simulink model "sampleModel2438_pp"  (R2018a)
settings: Solver=VariableStepAuto  StartTime=0.0  StopTime=10.0  RelTol=1e-3
undefined symbols (not defined in the file or in its folder): DiscIntNeverNeededParam, sigbuilder_block
libraries: simulink x299
(part 1 of 6)
settings Model: Creator=cyfuzz  LastModifiedBy=shafiul
settings CodeAppCC: StateflowObjectComments=on

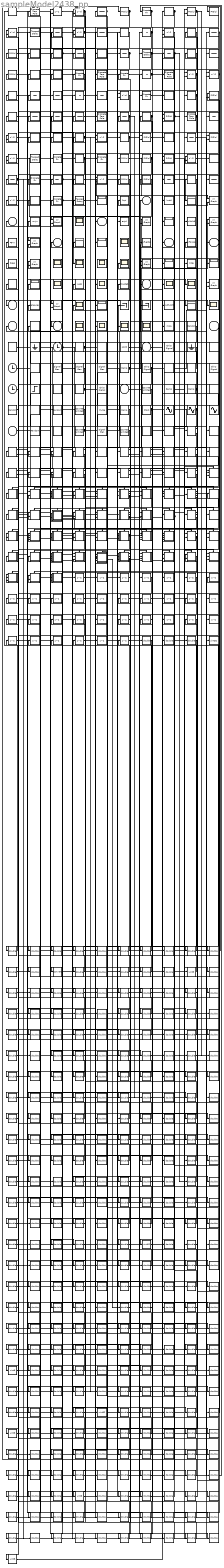
== system sampleModel2438_pp ==
  cfblk160 : Inport
  cfblk167 : Inport  Port=2
  cfblk186 : Inport  Port=3
  cfblk201 : Inport  Port=4
  cfblk{1,32,64,66,74,80,92} (7 alike) : simulink/Discrete/Transfer Fcn Real Zero  ZeroZ=0.75  ICPrevInput=0.0  DoSatur=off
      settings: SourceProductName=Simulink  SourceProductBaseCode=SL
  cfblk{6,10,21,31,76..77,86..87} (8 alike) : simulink/Continuous/PID Controller  Controller=PID  TimeDomain=Discrete-time  SampleTime=1  IntegratorMethod=Forward Euler  FilterMethod=Forward Euler  Form=Parallel  UseFilter=on  ControllerParametersSource=internal  P=1  I=1  D=0  N=100  InitialConditionSource=internal  InitialConditionForIntegrator=0  InitialConditionForFilter=0  ExternalReset=none  LimitOutput=off  UpperSaturationLimit=inf  LowerSaturationLimit=-inf  LinearizeAsGain=off  AntiWindupMode=none  Kb=1  TrackingMode=off  Kt=1  PParamMin=[]  PParamMax=[]  IParamMin=[]  IParamMax=[]  DParamMin=[]  DParamMax=[]  NParamMin=[]  NParamMax=[]  KbParamMin=[]  KbParamMax=[]  KtParamMin=[]  KtParamMax=[]  POutMin=[]  POutMax=[]  IOutMin=[]  IOutMax=[]  DOutMin=[]  DOutMax=[]  NOutMin=[]  NOutMax=[]  KbOutMin=[]  KbOutMax=[]  KtOutMin=[]  KtOutMax=[]  IntegratorOutMin=[]  IntegratorOutMax=[]  FilterOutMin=[]  FilterOutMax=[]  SumOutMin=[]  SumOutMax=[]  SumI1OutMin=[]  SumI1OutMax=[]  SumI2OutMin=[]  SumI2OutMax=[]  SumI3OutMin=[]  SumI3OutMax=[]  SumDOutMin=[]  SumDOutMax=[]  SaturationOutMin=[]  SaturationOutMax=[]  IntegratorContinuousStateAttributes=''  IntegratorStateMustResolveToSignalObject=off  IntegratorRTWStateStorageClass=Auto  FilterContinuousStateAttributes=''  FilterStateMustResolveToSignalObject=off  FilterRTWStateStorageClass=Auto  DifferentiatorICPrevScaledInput=0  DifferentiatorOutMin=[]  DifferentiatorOutMax=[]  FilterDiffOutCoefMin=[]  FilterDiffOutCoefMax=[]  SumDenOutMin=[]  SumDenOutMax=[]  SumNumOutMin=[]  SumNumOutMax=[]  ReciprocalOutMin=[]  ReciprocalOutMax=[]  DivideOutMin=[]  DivideOutMax=[]  TunerSelectOption=Transfer Function Based (PID Tuner App)
  cfblk{100,103,107,110,112,122,127,140,143} (9 alike) : simulink/Sinks/XY Graph  xmin=-1  xmax=1  ymin=-1  ymax=1  st=-1
  cfblk102 : ToFile  Filename=mvju  SaveFormat=Timeseries
  cfblk{104,116,123..126,133,135,138..139,144,150,154..157} (16 alike) : Scope
      cfblk104 settings: Floating=on
      cfblk116 settings: Floating=on
      cfblk123 settings: Floating=on
      cfblk125 settings: Floating=on
      cfblk133 settings: Floating=on
      cfblk154 settings: Floating=on
      cfblk157 settings: Floating=on
  cfblk106 : ToFile  Filename=eujd  SaveFormat=Timeseries
  cfblk{95,99,108,114..115,128,130,132,145,149} (10 alike) : Display
  cfblk109 : ToWorkspace  VariableName=xkbihtf  SaveFormat=Timeseries  SampleTime=-1
  cfblk11 : Delay  DelayLengthSource=Input port  SampleTime=1
      settings: InputPortMap=u0,p1
  cfblk111 : ToFile  Filename=cgvy  SaveFormat=Timeseries
  cfblk117 : ToWorkspace  VariableName=xfyezbp  SaveFormat=Timeseries  SampleTime=-1
  cfblk119 : ToWorkspace  VariableName=yrfonpq  SaveFormat=Timeseries  SampleTime=-1
  cfblk{12,27,72,94} (4 alike) : simulink/Discrete/Tapped Delay  vinit=0.0  samptime=-1  NumDelays=1  DelayOrder=Oldest  includeCurrent=off
  cfblk121 : ToFile  Filename=bcgq  SaveFormat=Timeseries
  cfblk129 : ToFile  Filename=mjtg  SaveFormat=Timeseries
  cfblk{13,15,20,43,52..53,56,81,90} (9 alike) : DiscreteTransferFcn  SampleTime=1
  cfblk131 : ToWorkspace  VariableName=whweswj  SaveFormat=Timeseries  SampleTime=-1
  cfblk134 : ToFile  Filename=jueb  SaveFormat=Timeseries
  cfblk136 : ToWorkspace  VariableName=tkwpteb  SaveFormat=Timeseries  SampleTime=-1
  cfblk{3,14,18,39..40,61,65,71,79,85} (10 alike) : Delay  ShowEnablePort=on  SampleTime=1
      settings: InputPortMap=u0,e6
  cfblk142 : ToWorkspace  VariableName=enguigy  SaveFormat=Timeseries  SampleTime=-1
  cfblk146 : Terminator
  cfblk147 : Terminator
  cfblk148 : ToWorkspace  VariableName=wdhubit  SaveFormat=Timeseries  SampleTime=-1
  cfblk152 : ToWorkspace  VariableName=eyoxfmy  SaveFormat=Timeseries  SampleTime=-1
  cfblk158 : ToFile  Filename=mojy  SaveFormat=Timeseries
  cfblk{159,191,193,202} (4 alike) : UniformRandomNumber  SampleTime=0.1
  cfblk16 : simulink/Discrete/Transfer Fcn Lead or Lag  PoleZ=0.95  ZeroZ=0.75  ICPrevOutput=0.0  ICPrevInput=0.0  DoSatur=off
      settings: SourceProductName=Simulink  SourceProductBaseCode=SL
  cfblk161 : simulink/Sources/Band-Limited White Noise  Cov=[0.1]  Ts=0.1  seed=[23341]
  cfblk162 : Ground
  cfblk163 : Clock
  cfblk164 : simulink/Sources/Band-Limited White Noise  Cov=[0.1]  Ts=0.1  seed=[23341]
  cfblk165 : Subsystem  Tag=STV Subsys  LoadFcn=sigbuilder_block('load');  StartFcn=sigbuilder_block('start');  StopFcn=sigbuilder_block('stop');  ClipboardFcn=sigbuilder_block('clipboard');  mask(Sigbuilder block){tuvar=[0:10]}
      mask help: Simulink:masks:SigbuilderBlock_MD
      mask init:
      | if ~strcmp(get_param(bdroot(gcbh),'SimulationStatus'),'stopped') tuvar = sigbuilder_block('maskInit'); end
      settings: CopyFcn=sigbuilder_block('copy');  DeleteFcn=sigbuilder_block('delete');  ModelCloseFcn=sigbuilder_block('modelClose');  PreSaveFcn=sigbuilder_block('preSave');  PauseFcn=sigbuilder_block('pause');  ContinueFcn=sigbuilder_block('continue');  NameChangeFcn=sigbuilder_block('namechange');  OpenFcn=sigbuilder_block('open',[437.6 199.2 550.4 400 ]);  CloseFcn=sigbuilder_block('close');
      mask Display: plot(0, 0, 100, 100,[2, 2, 32, 32, 2], [68, 8, 8, 68, 68],[32, 2], [38, 38], [32, 19, 2],[53, 60, 44], [32, 17, 17, 2],[16, 16, 31, 31]);txt = getActiveGroup(gcbh);text(2, 100, txt,'verticalAlignment', 'top');
  cfblk166 : Constant  Value=4120
  cfblk{168,177,180,185} (4 alike) : simulink/Sources/Chirp Signal  f1=0.1  T=100  f2=1
  cfblk169 : Ground
  cfblk17 : UnitDelay
  cfblk170 : Subsystem  Tag=STV Subsys  LoadFcn=sigbuilder_block('load');  StartFcn=sigbuilder_block('start');  StopFcn=sigbuilder_block('stop');  ClipboardFcn=sigbuilder_block('clipboard');  mask(Sigbuilder block){tuvar=[0:10]}
      mask help: Simulink:masks:SigbuilderBlock_MD
      mask init:
      | if ~strcmp(get_param(bdroot(gcbh),'SimulationStatus'),'stopped') tuvar = sigbuilder_block('maskInit'); end
      settings: CopyFcn=sigbuilder_block('copy');  DeleteFcn=sigbuilder_block('delete');  ModelCloseFcn=sigbuilder_block('modelClose');  PreSaveFcn=sigbuilder_block('preSave');  PauseFcn=sigbuilder_block('pause');  ContinueFcn=sigbuilder_block('continue');  NameChangeFcn=sigbuilder_block('namechange');  OpenFcn=sigbuilder_block('open',[437.6 199.2 550.4 400 ]);  CloseFcn=sigbuilder_block('close');
      mask Display: plot(0, 0, 100, 100,[2, 2, 32, 32, 2], [68, 8, 8, 68, 68],[32, 2], [38, 38], [32, 19, 2],[53, 60, 44], [32, 17, 17, 2],[16, 16, 31, 31]);txt = getActiveGroup(gcbh);text(2, 100, txt,'verticalAlignment', 'top');
  cfblk171 : Clock
  cfblk{172,178,190,192} (4 alike) : simulink/Sources/Repeating Sequence  rep_seq_t=[0 2]  rep_seq_y=[0 2]
  cfblk{173..175,205} (4 alike) : SignalGenerator  Units=rad/sec
  cfblk{176,188..189,196} (4 alike) : simulink/Sources/Ramp  slope=1  start=0  InitialOutput=0
  cfblk179 : Subsystem  Tag=STV Subsys  LoadFcn=sigbuilder_block('load');  StartFcn=sigbuilder_block('start');  StopFcn=sigbuilder_block('stop');  ClipboardFcn=sigbuilder_block('clipboard');  mask(Sigbuilder block){tuvar=[0:10]}
      mask help: Simulink:masks:SigbuilderBlock_MD
      mask init:
      | if ~strcmp(get_param(bdroot(gcbh),'SimulationStatus'),'stopped') tuvar = sigbuilder_block('maskInit'); end
      settings: CopyFcn=sigbuilder_block('copy');  DeleteFcn=sigbuilder_block('delete');  ModelCloseFcn=sigbuilder_block('modelClose');  PreSaveFcn=sigbuilder_block('preSave');  PauseFcn=sigbuilder_block('pause');  ContinueFcn=sigbuilder_block('continue');  NameChangeFcn=sigbuilder_block('namechange');  OpenFcn=sigbuilder_block('open',[437.6 199.2 550.4 400 ]);  CloseFcn=sigbuilder_block('close');
      mask Display: plot(0, 0, 100, 100,[2, 2, 32, 32, 2], [68, 8, 8, 68, 68],[32, 2], [38, 38], [32, 19, 2],[53, 60, 44], [32, 17, 17, 2],[16, 16, 31, 31]);txt = getActiveGroup(gcbh);text(2, 100, txt,'verticalAlignment', 'top');
  cfblk181 : Clock
  cfblk182 : Step  After=81  SampleTime=0
  cfblk183 : simulink/Sources/Repeating Sequence Stair  OutValues=[3 1 4 2 1].'  tsamp=-1  OutMin=[]  OutMax=[]  OutDataTypeStr=double  OutputDataTypeScalingMode=double  OutDataType=fixdt(0,8)  ConRadixGroup=Best Precision: Vector-wise  OutScaling=2^-12
  cfblk184 : simulink/Sources/Repeating Sequence Interpolated  OutValues=[3 1 4 2 1].'  TimeValues=[0 0.1 0.5 0.6 1].'  LookUpMeth=Interpolation-Use End Values  tsamp=0.01  OutMin=[]  OutMax=[]  OutDataTypeStr=double  OutputDataTypeScalingMode=double  OutDataType=fixdt(0,8)  OutScaling=2^-10
  cfblk{187,194,204,206} (4 alike) : simulink/Sources/Counter Limited  uplimit=7  tsamp=-1
  cfblk{8,19,23,48} (4 alike) : DiscreteStateSpace
  cfblk195 : DiscretePulseGenerator  PulseType=Time based  Period=10  PulseWidth=5
  cfblk197 : DigitalClock
  cfblk198 : Sin  SampleTime=0
  cfblk199 : Sin  SampleTime=0
  cfblk{2,35,38,55,59} (5 alike) : DiscreteZeroPole  Poles=[0 0.5]  Gain=1
  cfblk200 : Sin  SampleTime=0
  cfblk203 : simulink/Sources/Band-Limited White Noise  Cov=[0.1]  Ts=0.1  seed=[23341]
  cfblk207 : Subsystem  Tag=STV Subsys  LoadFcn=sigbuilder_block('load');  StartFcn=sigbuilder_block('start');  StopFcn=sigbuilder_block('stop');  ClipboardFcn=sigbuilder_block('clipboard');  mask(Sigbuilder block){tuvar=[0:10]}
      mask help: Simulink:masks:SigbuilderBlock_MD
      mask init:
      | if ~strcmp(get_param(bdroot(gcbh),'SimulationStatus'),'stopped') tuvar = sigbuilder_block('maskInit'); end
      settings: CopyFcn=sigbuilder_block('copy');  DeleteFcn=sigbuilder_block('delete');  ModelCloseFcn=sigbuilder_block('modelClose');  PreSaveFcn=sigbuilder_block('preSave');  PauseFcn=sigbuilder_block('pause');  ContinueFcn=sigbuilder_block('continue');  NameChangeFcn=sigbuilder_block('namechange');  OpenFcn=sigbuilder_block('open',[437.6 199.2 550.4 400 ]);  CloseFcn=sigbuilder_block('close');
      mask Display: plot(0, 0, 100, 100,[2, 2, 32, 32, 2], [68, 8, 8, 68, 68],[32, 2], [38, 38], [32, 19, 2],[53, 60, 44], [32, 17, 17, 2],[16, 16, 31, 31]);txt = getActiveGroup(gcbh);text(2, 100, txt,'verticalAlignment', 'top');
  cfblk{208..229} (22 alike) : If  SampleTime=1
  cfblk{22,33,63,89} (4 alike) : simulink/Discrete/Transfer Fcn First Order  PoleZ=0.95  ICPrevOutput=0.0  DoSatur=off
      settings: SourceProductName=Simulink
  cfblk230 : Subsystem  TreatAsAtomicUnit=on
  cfblk231 : Subsystem  TreatAsAtomicUnit=on
  cfblk232 : Subsystem  TreatAsAtomicUnit=on
  cfblk233 : Subsystem  TreatAsAtomicUnit=on
  cfblk234 : Subsystem  TreatAsAtomicUnit=on
  cfblk235 : Subsystem  TreatAsAtomicUnit=on
  cfblk236 : Subsystem  TreatAsAtomicUnit=on
  cfblk237 : Subsystem  TreatAsAtomicUnit=on
  cfblk238 : Subsystem  TreatAsAtomicUnit=on
  cfblk239 : Subsystem  TreatAsAtomicUnit=on
  cfblk{5,24,30,54} (4 alike) : DiscreteFilter  SampleTime=1
  cfblk240 : Subsystem  TreatAsAtomicUnit=on
  cfblk241 : Subsystem  TreatAsAtomicUnit=on
  cfblk242 : Subsystem  TreatAsAtomicUnit=on
  cfblk243 : Subsystem  TreatAsAtomicUnit=on
  cfblk244 : Subsystem  TreatAsAtomicUnit=on
  cfblk245 : Subsystem  TreatAsAtomicUnit=on
  cfblk246 : Subsystem  TreatAsAtomicUnit=on
  cfblk247 : Subsystem  TreatAsAtomicUnit=on
  cfblk248 : Subsystem  TreatAsAtomicUnit=on
  cfblk249 : Subsystem  TreatAsAtomicUnit=on
  cfblk{25,29,41,57,62,68,84} (7 alike) : simulink/Discrete/Difference  ICPrevInput=0.0  OutMin=[]  OutMax=[]  OutDataTypeStr=Inherit: Inherit via back propagation  OutDataType=fixdt(1, 16)  OutScaling=2^-10  DoSatur=off
  cfblk250 : Subsystem  TreatAsAtomicUnit=on
  cfblk251 : Subsystem  TreatAsAtomicUnit=on
  cfblk252 : Subsystem  TreatAsAtomicUnit=on
  cfblk253 : Subsystem  TreatAsAtomicUnit=on
  cfblk254 : Subsystem  TreatAsAtomicUnit=on
  cfblk255 : Subsystem  TreatAsAtomicUnit=on
  cfblk256 : Subsystem  TreatAsAtomicUnit=on
  cfblk257 : Subsystem  TreatAsAtomicUnit=on
  cfblk258 : Subsystem  TreatAsAtomicUnit=on
  cfblk259 : Subsystem  TreatAsAtomicUnit=on
  cfblk{26,28,42,45,60,69,83,88} (8 alike) : DiscreteIntegrator  ICPrevOutput=DiscIntNeverNeededParam  ICPrevScaledInput=DiscIntNeverNeededParam
  cfblk260 : Subsystem  TreatAsAtomicUnit=on
  cfblk261 : Subsystem  TreatAsAtomicUnit=on
  cfblk262 : Subsystem  TreatAsAtomicUnit=on
  cfblk263 : Subsystem  TreatAsAtomicUnit=on
  cfblk264 : Subsystem  TreatAsAtomicUnit=on
  cfblk265 : Subsystem  TreatAsAtomicUnit=on
  cfblk266 : Subsystem  TreatAsAtomicUnit=on
  cfblk267 : Subsystem  TreatAsAtomicUnit=on
  cfblk268 : Subsystem  TreatAsAtomicUnit=on
  cfblk269 : Subsystem  TreatAsAtomicUnit=on
  cfblk270 : Subsystem  TreatAsAtomicUnit=on
  cfblk271 : Subsystem  TreatAsAtomicUnit=on
  cfblk272 : Subsystem  TreatAsAtomicUnit=on
  cfblk273 : Subsystem  TreatAsAtomicUnit=on
  cfblk{91,274..306} (34 alike) : Delay  SampleTime=1
  cfblk307 : DataTypeConversion  OutDataTypeStr=double
  cfblk308 : DataTypeConversion  OutDataTypeStr=double
  cfblk309 : DataTypeConversion  OutDataTypeStr=double
  cfblk310 : DataTypeConversion  OutDataTypeStr=uint32
  cfblk{7,34,36,47,73,75,82,93} (8 alike) : DiscreteFir  SampleTime=1
  cfblk37 : UnitDelay
  cfblk4 : Delay  DelayLengthSource=Input port  SampleTime=1
      settings: InputPortMap=u0,p1
  cfblk44 : UnitDelay
  cfblk46 : Delay  DelayLengthSource=Input port  SampleTime=1
      settings: InputPortMap=u0,p1
  cfblk49 : simulink/Discrete/Transfer Fcn Lead or Lag  PoleZ=0.95  ZeroZ=0.75  ICPrevOutput=0.0  ICPrevInput=0.0  DoSatur=off
      settings: SourceProductName=Simulink  SourceProductBaseCode=SL
  cfblk{9,50,58,67,70,78} (6 alike) : simulink/Continuous/PID Controller (2DOF)  Controller=PID  TimeDomain=Discrete-time  SampleTime=1  IntegratorMethod=Forward Euler  FilterMethod=Forward Euler  Form=Parallel  UseFilter=on  ControllerParametersSource=internal  P=1  I=1  D=0  N=100  b=1  c=1  InitialConditionSource=internal  InitialConditionForIntegrator=0  InitialConditionForFilter=0  ExternalReset=none  LimitOutput=off  UpperSaturationLimit=inf  LowerSaturationLimit=-inf  LinearizeAsGain=off  AntiWindupMode=none  Kb=1  TrackingMode=off  Kt=1  PParamMin=[]  PParamMax=[]  IParamMin=[]  IParamMax=[]  DParamMin=[]  DParamMax=[]  NParamMin=[]  NParamMax=[]  bParamMin=[]  bParamMax=[]  cParamMin=[]  cParamMax=[]  KbParamMin=[]  KbParamMax=[]  KtParamMin=[]  KtParamMax=[]  POutMin=[]  POutMax=[]  IOutMin=[]  IOutMax=[]  DOutMin=[]  DOutMax=[]  NOutMin=[]  NOutMax=[]  bOutMin=[]  bOutMax=[]  cOutMin=[]  cOutMax=[]  KbOutMin=[]  KbOutMax=[]  KtOutMin=[]  KtOutMax=[]  IntegratorOutMin=[]  IntegratorOutMax=[]  FilterOutMin=[]  FilterOutMax=[]  SumOutMin=[]  SumOutMax=[]  Sum1OutMin=[]  Sum1OutMax=[]  Sum2OutMin=[]  Sum2OutMax=[]  Sum3OutMin=[]  Sum3OutMax=[]  SumI1OutMin=[]  SumI1OutMax=[]  SumI2OutMin=[]  SumI2OutMax=[]  SumI3OutMin=[]  SumI3OutMax=[]  SumDOutMin=[]  SumDOutMax=[]  SaturationOutMin=[]  SaturationOutMax=[]  IntegratorContinuousStateAttributes=''  IntegratorStateMustResolveToSignalObject=off  IntegratorRTWStateStorageClass=Auto  FilterContinuousStateAttributes=''  FilterStateMustResolveToSignalObject=off  FilterRTWStateStorageClass=Auto  DifferentiatorICPrevScaledInput=0  DifferentiatorOutMin=[]  DifferentiatorOutMax=[]  FilterDiffOutCoefMin=[]  FilterDiffOutCoefMax=[]  SumDenOutMin=[]  SumDenOutMax=[]  SumNumOutMin=[]  SumNumOutMax=[]  ReciprocalOutMin=[]  ReciprocalOutMax=[]  DivideOutMin=[]  DivideOutMax=[]  TunerSelectOption=Transfer Function Based (PID Tuner App)
  cfblk51 : simulink/Discrete/Transfer Fcn Lead or Lag  PoleZ=0.95  ZeroZ=0.75  ICPrevOutput=0.0  ICPrevInput=0.0  DoSatur=off
      settings: SourceProductName=Simulink  SourceProductBaseCode=SL
  cfblk96 : ToFile  Filename=fnpi  SaveFormat=Timeseries
  cfblk98 : ToFile  Filename=kudd  SaveFormat=Timeseries
  cyemi_{0..11,13..17,19..58,72,83..84,111..113,128..129,175..177,213..214,223..224,233..235,251,309..310,318,347..348,360..361,375..376,383..385,414,450..451,472,508,513..514,524..525,534..537,550..551,569..570,598..599,608..610,651..654,700..703,775..776,783..785,796,807,851..854,859..861,865..869,873..875,924..927,938,946..947,956..959,1005..1007,1014..1015,1026..1028,1037..1074,1076..1098,1100..1104,1106..1137,1139..1164} (283 alike) : DataTypeConversion  OutDataTypeStr=double
  cyemi_{18,1075,1105,1138,1165} (5 alike) : DataTypeConversion  OutDataTypeStr=uint8
  cyemi_1099 : DataTypeConversion  OutDataTypeStr=uint32
  cyemi_12 : DataTypeConversion  OutDataTypeStr=fixdt('ufix32_En8')
  cyemi_937 : DataTypeConversion  OutDataTypeStr=uint32
  cfblk97 : Outport
  cfblk101 : Outport  Port=2
  cfblk105 : Outport  Port=3
  cfblk113 : Outport  Port=4
  cfblk118 : Outport  Port=5
  cfblk120 : Outport  Port=6
  cfblk137 : Outport  Port=7
  cfblk141 : Outport  Port=8
  cfblk151 : Outport  Port=9
  cfblk153 : Outport  Port=10
  wires:
  cfblk10/1 -> cfblk135/1
  cfblk200/1 -> cfblk108/1
  cfblk83/1 -> cyemi_703/1, cyemi_1121/1
  cfblk58/1 -> cyemi_58/1, cyemi_1055/1, cyemi_1157/1
  cfblk45/1 -> cfblk145/1
  cfblk16/1 -> cfblk155/1
  cfblk4/1 -> cyemi_1058/1, cyemi_1155/1
  cfblk52/1 -> cfblk124/1
  cfblk23/1 -> cyemi_700/1, cyemi_1129/1
  cfblk189/1 -> cfblk118/1, cyemi_654/1, cyemi_1005/1
  cfblk195/1 -> cfblk97/1
  cfblk230/1(cfblk2) -> cfblk126/1, cyemi_1056/1
  cfblk176/1 -> cfblk107/1, cyemi_57/1
  cfblk15/1 -> cfblk147/1, cyemi_1113/1
  cfblk14/1 -> cyemi_29/1, cyemi_861/1
  cfblk77/1 -> cyemi_550/1, cyemi_1006/1
  cfblk199/1 -> cyemi_14/1, cyemi_234/1
  cfblk87/1 -> cfblk103/1
  cfblk62/1 -> cfblk149/1
  cfblk57/1 -> cfblk143/1, cyemi_3/1, cyemi_1057/1, cyemi_1125/1
  cfblk6/1 -> cfblk143/2, cfblk105/1
  cfblk244/1(cfblk2) -> cyemi_52/1, cyemi_1092/1
  cfblk55/1 -> cyemi_4/1, cyemi_1109/1
  cfblk84/1 -> cfblk100/1
  cfblk91/1 -> cfblk103/2
  cfblk24/1 -> cfblk112/1
  cfblk90/1 -> cfblk127/1
  cfblk8/1 -> cyemi_860/1, cyemi_1051/1
  cfblk197/1 -> cyemi_30/1, cyemi_1084/1
  cfblk59/1 -> cyemi_1079/1, cyemi_1096/1
  cfblk163/1 -> cyemi_41/1, cyemi_514/1
  cfblk20/1 -> cyemi_177/1, cyemi_785/1
  cfblk205/1 -> cfblk140/2, cyemi_1102/1
  cfblk204/1 -> cfblk146/1, cyemi_18/1, cyemi_1138/1
  cfblk86/1 -> cfblk141/1
  cfblk240/2(cfblk8) -> cyemi_869/1, cyemi_1073/1
  cfblk74/1 -> cyemi_55/1, cyemi_854/1
  cfblk28/1 -> cyemi_702/1, cyemi_1146/1
  cfblk66/1 -> cyemi_24/1, cyemi_1163/1
  cfblk177/1 -> cyemi_1/1, cyemi_1043/1
  cfblk40/1 -> cyemi_49/1, cyemi_1074/1
  cfblk250/1(cfblk2) -> cfblk128/1
  cfblk246/3(cfblk10) -> cfblk138/1, cyemi_1070/1
  cfblk255/1(cfblk2) -> cfblk101/1
  cfblk11/1 -> cfblk139/1
  cfblk261/2(cfblk11) -> cyemi_957/1, cyemi_1156/1
  cfblk256/1(cfblk2) -> cfblk110/1, cyemi_1135/1
  cfblk182/1 -> cfblk112/2
  cfblk264/1(cfblk2) -> cfblk114/1
  cfblk257/1(cfblk2) -> cfblk151/1, cyemi_36/1
  cfblk81/1 -> cyemi_21/1, cyemi_25/1
  cfblk27/1 -> cyemi_385/1, cyemi_958/1
  cfblk85/1 -> cfblk156/1
  cfblk37/1 -> cfblk150/1, cyemi_1015/1
  cfblk248/2(cfblk11) -> cyemi_1067/1, cyemi_1077/1
  cfblk12/1 -> cfblk95/1
  cfblk93/1 -> cfblk107/2, cyemi_701/1
  cfblk201/1 -> cfblk120/1
  cfblk71/1 -> cfblk115/1
  cfblk64/1 -> cyemi_5/1, cyemi_1089/1
  cfblk259/2(cfblk8) -> cyemi_213/1, cyemi_938/1
  cfblk5/1 -> cyemi_536/1, cyemi_1068/1
  cfblk245/1(cfblk2) -> cfblk122/1, cyemi_853/1
  cfblk184/1 -> cfblk130/1, cyemi_27/1, cyemi_43/1
  cfblk232/1(cfblk2) -> cyemi_1090/1, cyemi_1143/1
  cfblk179/1(Signal 1) -> cfblk132/1
  cfblk48/1 -> cfblk122/2
  cfblk160/1 -> cyemi_214/1, cyemi_867/1
  cfblk76/1 -> cfblk99/1
  cfblk26/1 -> cyemi_472/1, cyemi_959/1
  cfblk7/1 -> cyemi_44/1, cyemi_610/1
  cfblk39/1 -> cfblk127/2, cyemi_1119/1
  cfblk49/1 -> cyemi_53/1, cyemi_537/1
  cfblk88/1 -> cfblk110/2
  cfblk9/1 -> cyemi_72/1, cyemi_1053/1
  cfblk265/2(cfblk10) -> cyemi_1049/1, cyemi_1050/1
  cfblk162/1 -> cyemi_54/1, cyemi_383/1
  cfblk272/1(cfblk2) -> cyemi_513/1, cyemi_868/1
  cfblk203/1 -> cfblk113/1
  cfblk17/1 -> cyemi_551/1, cyemi_926/1
  cfblk238/2(cfblk17) -> cfblk100/2
  cfblk164/1 -> cyemi_1080/1, cyemi_1152/1
  cfblk235/2(cfblk12) -> cfblk144/1
  cfblk44/1 -> cfblk137/1
  cfblk56/1 -> cfblk153/1, cyemi_235/1
  cfblk266/3(cfblk16) -> cyemi_1054/1, cyemi_1118/1
  cfblk260/3(cfblk15) -> cyemi_26/1, cyemi_1145/1
  cfblk178/1 -> cfblk140/1
  cfblk170/1(Signal 1) -> cyemi_6/1, cyemi_23/1, cyemi_28/1
  cfblk234/3(cfblk15) -> cyemi_1039/1, cyemi_1101/1
  cfblk236/3(cfblk12) -> cyemi_1088/1, cyemi_1103/1
  cfblk208/1 -> cfblk230/Action
  cfblk208/2 -> cfblk231/Action
  cfblk209/1 -> cfblk232/Action
  cfblk209/2 -> cfblk233/Action
  cfblk210/1 -> cfblk234/Action
  cfblk210/2 -> cfblk235/Action
  cfblk211/1 -> cfblk236/Action
  cfblk211/2 -> cfblk237/Action
  cfblk212/1 -> cfblk238/Action
  cfblk212/2 -> cfblk239/Action
  cfblk213/1 -> cfblk240/Action
  cfblk213/2 -> cfblk241/Action
  cfblk214/1 -> cfblk242/Action
  cfblk214/2 -> cfblk243/Action
  cfblk215/1 -> cfblk244/Action
  cfblk215/2 -> cfblk245/Action
  cfblk216/1 -> cfblk246/Action
  cfblk216/2 -> cfblk247/Action
  cfblk217/1 -> cfblk248/Action
  cfblk217/2 -> cfblk249/Action
  cfblk218/1 -> cfblk250/Action
  cfblk218/2 -> cfblk251/Action
  cfblk219/1 -> cfblk252/Action
  cfblk219/2 -> cfblk253/Action
  cfblk220/1 -> cfblk254/Action
  cfblk220/2 -> cfblk255/Action
  cfblk221/1 -> cfblk256/Action
  cfblk221/2 -> cfblk257/Action
  cfblk222/1 -> cfblk258/Action
  cfblk222/2 -> cfblk259/Action
  cfblk223/1 -> cfblk260/Action
  cfblk223/2 -> cfblk261/Action
  cfblk224/1 -> cfblk262/Action
  cfblk224/2 -> cfblk263/Action
  cfblk225/1 -> cfblk264/Action
  cfblk225/2 -> cfblk265/Action
  cfblk226/1 -> cfblk266/Action
  cfblk226/2 -> cfblk267/Action
  cfblk227/1 -> cfblk268/Action
  cfblk227/2 -> cfblk269/Action
  cfblk228/1 -> cfblk270/Action
  cfblk228/2 -> cfblk271/Action
  cfblk229/1 -> cfblk272/Action
  cfblk229/2 -> cfblk273/Action
  cyemi_0/1 -> cfblk1/1
  cfblk283/1 -> cyemi_0/1
  cyemi_1/1 -> cfblk10/1
  cyemi_2/1 -> cfblk102/1
  cfblk249/2(cfblk6) -> cyemi_2/1
  cyemi_3/1 -> cfblk106/1
  cyemi_4/1 -> cfblk109/1
  cyemi_5/1 -> cfblk11/1
  cyemi_6/1 -> cfblk11/2
  cyemi_7/1 -> cfblk111/1
  cfblk65/1 -> cyemi_7/1
  cyemi_8/1 -> cfblk117/1
  cfblk53/1 -> cyemi_8/1
  cyemi_9/1 -> cfblk119/1
  cfblk72/1 -> cyemi_9/1
  cyemi_10/1 -> cfblk12/1
  cfblk18/1 -> cyemi_10/1
  cyemi_11/1 -> cfblk121/1
  cfblk60/1 -> cyemi_11/1
  cyemi_12/1 -> cfblk129/1
  cfblk75/1 -> cyemi_12/1
  cyemi_13/1 -> cfblk13/1
  cfblk247/2(cfblk16) -> cyemi_13/1
  cyemi_14/1 -> cfblk131/1
  cyemi_15/1 -> cfblk134/1
  cfblk173/1 -> cyemi_15/1
  cyemi_16/1 -> cfblk136/1
  cfblk190/1 -> cyemi_16/1
  cyemi_17/1 -> cfblk14/1
  cfblk238/1(cfblk2) -> cyemi_17/1
  cyemi_18/1 -> cfblk14/2
  cyemi_19/1 -> cfblk142/1
  cfblk248/1(cfblk2) -> cyemi_19/1
  cyemi_20/1 -> cfblk148/1
  cfblk181/1 -> cyemi_20/1
  cyemi_21/1 -> cfblk15/1
  cyemi_22/1 -> cfblk152/1
  cfblk263/2(cfblk8) -> cyemi_22/1
  cyemi_23/1 -> cfblk158/1
  cyemi_24/1 -> cfblk16/1
  cyemi_25/1 -> cfblk17/1
  cyemi_26/1 -> cfblk18/1
  cyemi_27/1 -> cfblk18/2
  cyemi_28/1 -> cfblk19/1
  cyemi_29/1 -> cfblk2/1
  cyemi_30/1 -> cfblk20/1
  cyemi_31/1 -> cfblk208/1
  cfblk295/1 -> cyemi_31/1
  cyemi_32/1 -> cfblk209/1
  cfblk294/1 -> cyemi_32/1
  cyemi_33/1 -> cfblk21/1
  cfblk161/1 -> cyemi_33/1
  cyemi_34/1 -> cfblk210/1
  cfblk261/1(cfblk2) -> cyemi_34/1
  cyemi_35/1 -> cfblk211/1
  cfblk300/1 -> cyemi_35/1
  cyemi_36/1 -> cfblk212/1
  cyemi_37/1 -> cfblk213/1
  cfblk167/1 -> cyemi_37/1
  cyemi_38/1 -> cfblk214/1
  cfblk287/1 -> cyemi_38/1
  cyemi_39/1 -> cfblk215/1
  cfblk69/1 -> cyemi_39/1
  cyemi_40/1 -> cfblk216/1
  cfblk240/1(cfblk2) -> cyemi_40/1
  cyemi_41/1 -> cfblk217/1
  cyemi_42/1 -> cfblk218/1
  cfblk196/1 -> cyemi_42/1
  cyemi_43/1 -> cfblk219/1
  cyemi_44/1 -> cfblk22/1
  cyemi_45/1 -> cfblk220/1
  cfblk233/1(cfblk2) -> cyemi_45/1
  cyemi_46/1 -> cfblk221/1
  cfblk236/1(cfblk2) -> cyemi_46/1
  cyemi_47/1 -> cfblk222/1
  cfblk299/1 -> cyemi_47/1
  cyemi_48/1 -> cfblk223/1
  cfblk288/1 -> cyemi_48/1
  cyemi_49/1 -> cfblk224/1
  cyemi_50/1 -> cfblk225/1
  cfblk80/1 -> cyemi_50/1
  cyemi_51/1 -> cfblk226/1
  cfblk1/1 -> cyemi_51/1
  cyemi_52/1 -> cfblk227/1
  cyemi_53/1 -> cfblk228/1
  cyemi_54/1 -> cfblk229/1
  cyemi_55/1 -> cfblk23/1
  cyemi_56/1 -> cfblk230/1(cfblk1)
  cfblk242/2(cfblk10) -> cyemi_56/1
  cyemi_57/1 -> cfblk230/2(cfblk13)
  cyemi_58/1 -> cfblk230/3(cfblk14)
  cyemi_72/1 -> cfblk231/1(cfblk1)
  cyemi_83/1 -> cfblk232/1(cfblk1)
  cfblk277/1 -> cyemi_83/1
  cyemi_84/1 -> cfblk232/2(cfblk8)
  cfblk262/1(cfblk2) -> cyemi_84/1
  cyemi_111/1 -> cfblk233/1(cfblk1)
  cfblk298/1 -> cyemi_111/1
  cyemi_112/1 -> cfblk233/2(cfblk13)
  cfblk165/1(Signal 1) -> cyemi_112/1
  cyemi_113/1 -> cfblk233/3(cfblk14)
  cfblk274/1 -> cyemi_113/1
  cyemi_128/1 -> cfblk234/1(cfblk1)
  cfblk270/1(cfblk2) -> cyemi_128/1
  cyemi_129/1 -> cfblk234/2(cfblk13)
  cfblk251/1(cfblk2) -> cyemi_129/1
  cyemi_175/1 -> cfblk235/1(cfblk1)
  cfblk186/1 -> cyemi_175/1
  cyemi_176/1 -> cfblk235/2(cfblk10)
  cfblk36/1 -> cyemi_176/1
  cyemi_177/1 -> cfblk235/3(cfblk11)
  cyemi_213/1 -> cfblk236/1(cfblk1)
  cyemi_214/1 -> cfblk236/2(cfblk10)
  cyemi_223/1 -> cfblk237/1(cfblk1)
  cfblk236/2(cfblk11) -> cyemi_223/1
  cyemi_224/1 -> cfblk237/2(cfblk9)
  cfblk234/2(cfblk14) -> cyemi_224/1
  cyemi_233/1 -> cfblk238/1(cfblk1)
  cfblk61/1 -> cyemi_233/1
  cyemi_234/1 -> cfblk238/2(cfblk15)
  cyemi_235/1 -> cfblk238/3(cfblk16)
  cyemi_251/1 -> cfblk239/1(cfblk1)
  cfblk291/1 -> cyemi_251/1
  cyemi_309/1 -> cfblk24/1
  cfblk32/1 -> cyemi_309/1
  cyemi_310/1 -> cfblk240/1(cfblk1)
  cfblk79/1 -> cyemi_310/1
  cyemi_318/1 -> cfblk241/1(cfblk1)
  cfblk50/1 -> cyemi_318/1
  cyemi_347/1 -> cfblk242/1(cfblk1)
  cfblk278/1 -> cyemi_347/1
  cyemi_348/1 -> cfblk242/2(cfblk9)
  cfblk259/1(cfblk2) -> cyemi_348/1
  cyemi_360/1 -> cfblk243/1(cfblk1)
  cfblk293/1 -> cyemi_360/1
  cyemi_361/1 -> cfblk243/2(cfblk13)
  cfblk280/1 -> cyemi_361/1
  cyemi_375/1 -> cfblk244/1(cfblk1)
  cfblk275/1 -> cyemi_375/1
  cyemi_376/1 -> cfblk244/2(cfblk7)
  cfblk290/1 -> cyemi_376/1
  cyemi_383/1 -> cfblk245/1(cfblk1)
  cyemi_384/1 -> cfblk245/2(cfblk8)
  cfblk306/1 -> cyemi_384/1
  cyemi_385/1 -> cfblk245/3(cfblk9)
  cyemi_414/1 -> cfblk246/1(cfblk1)
  cfblk292/1 -> cyemi_414/1
  cyemi_450/1 -> cfblk247/1(cfblk1)
  cfblk185/1 -> cyemi_450/1
  cyemi_451/1 -> cfblk247/2(cfblk15)
  cfblk266/2(cfblk15) -> cyemi_451/1
  cyemi_472/1 -> cfblk248/1(cfblk1)
  cyemi_508/1 -> cfblk249/1(cfblk1)
  cfblk302/1 -> cyemi_508/1
  cyemi_513/1 -> cfblk25/1
  cyemi_514/1 -> cfblk250/1(cfblk1)
  cyemi_524/1 -> cfblk251/1(cfblk1)
  cfblk254/1(cfblk2) -> cyemi_524/1
  cyemi_525/1 -> cfblk251/2(cfblk9)
  cfblk67/1 -> cyemi_525/1
  cyemi_534/1 -> cfblk252/1(cfblk1)
  cfblk73/1 -> cyemi_534/1
  cyemi_535/1 -> cfblk252/2(cfblk12)
  cfblk268/1(cfblk2) -> cyemi_535/1
  cyemi_536/1 -> cfblk252/3(cfblk13)
  cyemi_537/1 -> cfblk252/4(cfblk14)
  cyemi_550/1 -> cfblk253/1(cfblk1)
  cyemi_551/1 -> cfblk253/2(cfblk15)
  cyemi_569/1 -> cfblk254/1(cfblk1)
  cfblk296/1 -> cyemi_569/1
  cyemi_570/1 -> cfblk254/2(cfblk11)
  cfblk297/1 -> cyemi_570/1
  cyemi_598/1 -> cfblk255/1(cfblk1)
  cfblk193/1 -> cyemi_598/1
  cyemi_599/1 -> cfblk255/2(cfblk8)
  cfblk188/1 -> cyemi_599/1
  cyemi_608/1 -> cfblk256/1(cfblk1)
  cfblk254/2(cfblk12) -> cyemi_608/1
  cyemi_609/1 -> cfblk256/2(cfblk16)
  cfblk271/1(cfblk2) -> cyemi_609/1
  cyemi_610/1 -> cfblk256/3(cfblk17)
  cyemi_651/1 -> cfblk257/1(cfblk1)
  cfblk202/1 -> cyemi_651/1
  cyemi_652/1 -> cfblk257/2(cfblk15)
  cfblk169/1 -> cyemi_652/1
  cyemi_653/1 -> cfblk257/3(cfblk16)
  cfblk243/4(cfblk16) -> cyemi_653/1
  cyemi_654/1 -> cfblk257/4(cfblk17)
  cyemi_700/1 -> cfblk258/1(cfblk1)
  cyemi_701/1 -> cfblk258/2(cfblk13)
  cyemi_702/1 -> cfblk258/3(cfblk14)
  cyemi_703/1 -> cfblk258/4(cfblk15)
  cyemi_775/1 -> cfblk259/1(cfblk1)
  cfblk246/1(cfblk2) -> cyemi_775/1
  cyemi_776/1 -> cfblk259/2(cfblk7)
  cfblk279/1 -> cyemi_776/1
  cyemi_783/1 -> cfblk26/1
  cfblk266/1(cfblk2) -> cyemi_783/1
  cyemi_784/1 -> cfblk260/1(cfblk1)
  cfblk258/1(cfblk2) -> cyemi_784/1
  cyemi_785/1 -> cfblk260/2(cfblk13)
  cyemi_796/1 -> cfblk261/1(cfblk1)
  cfblk43/1 -> cyemi_796/1
  cyemi_807/1 -> cfblk262/1(cfblk1)
  cfblk301/1 -> cyemi_807/1
  cyemi_851/1 -> cfblk263/1(cfblk1)
  cfblk29/1 -> cyemi_851/1
  cyemi_852/1 -> cfblk263/2(cfblk5)
  cfblk308/1 -> cyemi_852/1
  cyemi_853/1 -> cfblk263/3(cfblk6)
  cyemi_854/1 -> cfblk263/4(cfblk7)
  cyemi_859/1 -> cfblk264/1(cfblk1)
  cfblk31/1 -> cyemi_859/1
  cyemi_860/1 -> cfblk264/2(cfblk6)
  cyemi_861/1 -> cfblk264/3(cfblk7)
  cyemi_865/1 -> cfblk265/1(cfblk1)
  cfblk260/2(cfblk14) -> cyemi_865/1
  cyemi_866/1 -> cfblk265/2(cfblk6)
  cfblk241/1(cfblk2) -> cyemi_866/1
  cyemi_867/1 -> cfblk265/3(cfblk7)
  cyemi_868/1 -> cfblk265/4(cfblk8)
  cyemi_869/1 -> cfblk265/5(cfblk9)
  cyemi_873/1 -> cfblk266/1(cfblk1)
  cfblk305/1 -> cyemi_873/1
  cyemi_874/1 -> cfblk266/2(cfblk13)
  cfblk285/1 -> cyemi_874/1
  cyemi_875/1 -> cfblk266/3(cfblk14)
  cfblk281/1 -> cyemi_875/1
  cyemi_924/1 -> cfblk267/1(cfblk1)
  cfblk303/1 -> cyemi_924/1
  cyemi_925/1 -> cfblk267/2(cfblk10)
  cfblk282/1 -> cyemi_925/1
  cyemi_926/1 -> cfblk267/3(cfblk11)
  cyemi_927/1 -> cfblk267/4(cfblk12)
  cfblk276/1 -> cyemi_927/1
  cyemi_937/1 -> cfblk268/1(cfblk1)
  cfblk239/4(cfblk16) -> cyemi_937/1
  cyemi_938/1 -> cfblk268/2(cfblk7)
  cyemi_946/1 -> cfblk269/1(cfblk1)
  cfblk166/1 -> cyemi_946/1
  cyemi_947/1 -> cfblk269/2(cfblk10)
  cfblk175/1 -> cyemi_947/1
  cyemi_956/1 -> cfblk27/1
  cfblk191/1 -> cyemi_956/1
  cyemi_957/1 -> cfblk270/1(cfblk1)
  cyemi_958/1 -> cfblk270/2(cfblk9)
  cyemi_959/1 -> cfblk270/3(cfblk10)
  cyemi_1005/1 -> cfblk271/1(cfblk1)
  cyemi_1006/1 -> cfblk271/2(cfblk8)
  cyemi_1007/1 -> cfblk271/3(cfblk9)
  cfblk286/1 -> cyemi_1007/1
  cyemi_1014/1 -> cfblk272/1(cfblk1)
  cfblk241/3(cfblk8) -> cyemi_1014/1
  cyemi_1015/1 -> cfblk272/2(cfblk10)
  cyemi_1026/1 -> cfblk273/1(cfblk1)
  cfblk284/1 -> cyemi_1026/1
  cyemi_1027/1 -> cfblk273/2(cfblk9)
  cfblk255/2(cfblk9) -> cyemi_1027/1
  cyemi_1028/1 -> cfblk273/3(cfblk10)
  cfblk289/1 -> cyemi_1028/1
  cyemi_1037/1 -> cfblk274/1
  cfblk242/1(cfblk2) -> cyemi_1037/1
  cyemi_1038/1 -> cfblk275/1
  cfblk22/1 -> cyemi_1038/1
  cyemi_1039/1 -> cfblk276/1
  cyemi_1040/1 -> cfblk277/1
  cfblk267/1(cfblk2) -> cyemi_1040/1
  cyemi_1041/1 -> cfblk278/1
  cfblk3/1 -> cyemi_1041/1
  cyemi_1042/1 -> cfblk279/1
  cfblk267/3(cfblk14) -> cyemi_1042/1
  cyemi_1043/1 -> cfblk28/1
  cyemi_1044/1 -> cfblk280/1
  cfblk25/1 -> cyemi_1044/1
  cyemi_1045/1 -> cfblk281/1
  cfblk243/1(cfblk2) -> cyemi_1045/1
  cyemi_1046/1 -> cfblk282/1
  cfblk235/1(cfblk2) -> cyemi_1046/1
  cyemi_1047/1 -> cfblk283/1
  cfblk260/1(cfblk2) -> cyemi_1047/1
  cyemi_1048/1 -> cfblk284/1
  cfblk70/1 -> cyemi_1048/1
  cyemi_1049/1 -> cfblk285/1
  cyemi_1050/1 -> cfblk286/1
  cyemi_1051/1 -> cfblk287/1
  cyemi_1052/1 -> cfblk288/1
  cfblk82/1 -> cyemi_1052/1
  cyemi_1053/1 -> cfblk289/1
  cyemi_1054/1 -> cfblk29/1
  cyemi_1055/1 -> cfblk290/1
  cyemi_1056/1 -> cfblk291/1
  cyemi_1057/1 -> cfblk292/1
  cyemi_1058/1 -> cfblk293/1
  cyemi_1059/1 -> cfblk294/1
  cfblk239/3(cfblk15) -> cyemi_1059/1
  cyemi_1060/1 -> cfblk295/1
  cfblk252/2(cfblk15) -> cyemi_1060/1
  cyemi_1061/1 -> cfblk296/1
  cfblk268/2(cfblk8) -> cyemi_1061/1
  cyemi_1062/1 -> cfblk297/1
  cfblk41/1 -> cyemi_1062/1
  cyemi_1063/1 -> cfblk298/1
  cfblk47/1 -> cyemi_1063/1
  cyemi_1064/1 -> cfblk299/1
  cfblk42/1 -> cyemi_1064/1
  cyemi_1065/1 -> cfblk3/1
  cfblk174/1 -> cyemi_1065/1
  cyemi_1066/1 -> cfblk3/2
  cfblk267/2(cfblk13) -> cyemi_1066/1
  cyemi_1067/1 -> cfblk30/1
  cyemi_1068/1 -> cfblk300/1
  cyemi_1069/1 -> cfblk301/1
  cfblk246/2(cfblk9) -> cyemi_1069/1
  cyemi_1070/1 -> cfblk302/1
  cyemi_1071/1 -> cfblk303/1
  cfblk253/2(cfblk16) -> cyemi_1071/1
  cyemi_1072/1 -> cfblk304/1
  cfblk247/3(cfblk17) -> cyemi_1072/1
  cyemi_1073/1 -> cfblk305/1
  cyemi_1074/1 -> cfblk306/1
  cyemi_1075/1 -> cfblk307/1
  cfblk187/1 -> cyemi_1075/1
  cyemi_1076/1 -> cfblk308/1
  cfblk46/1 -> cyemi_1076/1
  cyemi_1077/1 -> cfblk309/1
  cyemi_1078/1 -> cfblk31/1
  cfblk249/1(cfblk2) -> cyemi_1078/1
  cyemi_1079/1 -> cfblk310/1
  cyemi_1080/1 -> cfblk32/1
  cyemi_1081/1 -> cfblk33/1
  cfblk255/3(cfblk10) -> cyemi_1081/1
  cyemi_1082/1 -> cfblk34/1
  cfblk250/2(cfblk10) -> cyemi_1082/1
  cyemi_1083/1 -> cfblk35/1
  cfblk243/5(cfblk17) -> cyemi_1083/1
  cyemi_1084/1 -> cfblk36/1
  cyemi_1085/1 -> cfblk37/1
  cfblk254/3(cfblk13) -> cyemi_1085/1
  cyemi_1086/1 -> cfblk38/1
  cfblk249/3(cfblk7) -> cyemi_1086/1
  cyemi_1087/1 -> cfblk39/1
  cfblk183/1 -> cyemi_1087/1
  cyemi_1088/1 -> cfblk39/2
  cyemi_1089/1 -> cfblk4/1
  cyemi_1090/1 -> cfblk4/2
  cyemi_1091/1 -> cfblk40/1
  cfblk51/1 -> cyemi_1091/1
  cyemi_1092/1 -> cfblk40/2
  cyemi_1093/1 -> cfblk41/1
  cfblk35/1 -> cyemi_1093/1
  cyemi_1094/1 -> cfblk42/1
  cfblk78/1 -> cyemi_1094/1
  cyemi_1095/1 -> cfblk43/1
  cfblk243/2(cfblk14) -> cyemi_1095/1
  cyemi_1096/1 -> cfblk44/1
  cyemi_1097/1 -> cfblk45/1
  cfblk68/1 -> cyemi_1097/1
  cyemi_1098/1 -> cfblk46/1
  cfblk309/1 -> cyemi_1098/1
  cyemi_1099/1 -> cfblk46/2
  cfblk310/1 -> cyemi_1099/1
  cyemi_1100/1 -> cfblk47/1
  cfblk33/1 -> cyemi_1100/1
  cyemi_1101/1 -> cfblk48/1
  cyemi_1102/1 -> cfblk49/1
  cyemi_1103/1 -> cfblk5/1
  cyemi_1104/1 -> cfblk50/1
  cfblk198/1 -> cyemi_1104/1
  cyemi_1105/1 -> cfblk50/2
  cfblk194/1 -> cyemi_1105/1
  cyemi_1106/1 -> cfblk51/1
  cfblk172/1 -> cyemi_1106/1
  cyemi_1107/1 -> cfblk52/1
  cfblk180/1 -> cyemi_1107/1
  cyemi_1108/1 -> cfblk53/1
  cfblk263/3(cfblk9) -> cyemi_1108/1
  cyemi_1109/1 -> cfblk54/1
  cyemi_1110/1 -> cfblk55/1
  cfblk237/1(cfblk2) -> cyemi_1110/1
  cyemi_1111/1 -> cfblk56/1
  cfblk263/1(cfblk2) -> cyemi_1111/1
  cyemi_1112/1 -> cfblk57/1
  cfblk239/1(cfblk2) -> cyemi_1112/1
  cyemi_1113/1 -> cfblk58/1
  cyemi_1114/1 -> cfblk58/2
  cfblk2/1 -> cyemi_1114/1
  cyemi_1115/1 -> cfblk59/1
  cfblk307/1 -> cyemi_1115/1
  cyemi_1116/1 -> cfblk6/1
  cfblk21/1 -> cyemi_1116/1
  cyemi_1117/1 -> cfblk60/1
  cfblk34/1 -> cyemi_1117/1
  cyemi_1118/1 -> cfblk61/1
  cyemi_1119/1 -> cfblk61/2
  cyemi_1120/1 -> cfblk62/1
  cfblk237/2(cfblk10) -> cyemi_1120/1
  cyemi_1121/1 -> cfblk63/1
  cyemi_1122/1 -> cfblk64/1
  cfblk94/1 -> cyemi_1122/1
  cyemi_1123/1 -> cfblk65/1
  cfblk207/1(Signal 1) -> cyemi_1123/1
  cyemi_1124/1 -> cfblk65/2
  cfblk243/3(cfblk15) -> cyemi_1124/1
  cyemi_1125/1 -> cfblk66/1
  cyemi_1126/1 -> cfblk67/1
  cfblk252/1(cfblk2) -> cyemi_1126/1
  cyemi_1127/1 -> cfblk67/2
  cfblk241/2(cfblk7) -> cyemi_1127/1
  cyemi_1128/1 -> cfblk68/1
  cfblk19/1 -> cyemi_1128/1
  cyemi_1129/1 -> cfblk69/1
  cyemi_1130/1 -> cfblk7/1
  cfblk234/1(cfblk2) -> cyemi_1130/1
  cyemi_1131/1 -> cfblk70/1
  cfblk265/1(cfblk2) -> cyemi_1131/1
  cyemi_1132/1 -> cfblk70/2
  cfblk159/1 -> cyemi_1132/1
  cyemi_1133/1 -> cfblk71/1
  cfblk273/1(cfblk2) -> cyemi_1133/1
  cyemi_1134/1 -> cfblk71/2
  cfblk239/2(cfblk14) -> cyemi_1134/1
  cyemi_1135/1 -> cfblk72/1
  cyemi_1136/1 -> cfblk73/1
  cfblk269/1(cfblk2) -> cyemi_1136/1
  cyemi_1137/1 -> cfblk74/1
  cfblk30/1 -> cyemi_1137/1
  cyemi_1138/1 -> cfblk75/1
  cyemi_1139/1 -> cfblk76/1
  cfblk171/1 -> cyemi_1139/1
  cyemi_1140/1 -> cfblk77/1
  cfblk247/1(cfblk2) -> cyemi_1140/1
  cyemi_1141/1 -> cfblk78/1
  cfblk38/1 -> cyemi_1141/1
  cyemi_1142/1 -> cfblk78/2
  cfblk233/2(cfblk15) -> cyemi_1142/1
  cyemi_1143/1 -> cfblk79/1
  cyemi_1144/1 -> cfblk79/2
  cfblk304/1 -> cyemi_1144/1
  cyemi_1145/1 -> cfblk8/1
  cyemi_1146/1 -> cfblk80/1
  cyemi_1147/1 -> cfblk81/1
  cfblk168/1 -> cyemi_1147/1
  cyemi_1148/1 -> cfblk82/1
  cfblk270/2(cfblk11) -> cyemi_1148/1
  cyemi_1149/1 -> cfblk83/1
  cfblk192/1 -> cyemi_1149/1
  cyemi_1150/1 -> cfblk84/1
  cfblk54/1 -> cyemi_1150/1
  cyemi_1151/1 -> cfblk85/1
  cfblk253/3(cfblk17) -> cyemi_1151/1
  cyemi_1152/1 -> cfblk85/2
  cyemi_1153/1 -> cfblk86/1
  cfblk13/1 -> cyemi_1153/1
  cyemi_1154/1 -> cfblk87/1
  cfblk231/1(cfblk2) -> cyemi_1154/1
  cyemi_1155/1 -> cfblk88/1
  cyemi_1156/1 -> cfblk89/1
  cyemi_1157/1 -> cfblk9/1
  cyemi_1158/1 -> cfblk9/2
  cfblk63/1 -> cyemi_1158/1
  cyemi_1159/1 -> cfblk90/1
  cfblk253/1(cfblk2) -> cyemi_1159/1
  cyemi_1160/1 -> cfblk91/1
  cfblk89/1 -> cyemi_1160/1
  cyemi_1161/1 -> cfblk92/1
  cfblk270/3(cfblk12) -> cyemi_1161/1
  cyemi_1162/1 -> cfblk93/1
  cfblk262/2(cfblk7) -> cyemi_1162/1
  cyemi_1163/1 -> cfblk94/1
  cyemi_1164/1 -> cfblk96/1
  cfblk92/1 -> cyemi_1164/1
  cyemi_1165/1 -> cfblk98/1
  cfblk206/1 -> cyemi_1165/1

== system sampleModel2438_pp/cfblk165 ==
  Demux : Demux  Tag=STV Demux  Outputs=1
  FromWs : FromWorkspace  Tag=STV FromWs  VariableName=tuvar  SampleTime=0
      SigBuilderData=|
      | common.afterFinalStr = 'Extrapolate'
      | common.sampleTime = 0
      | dataSet.timeRange = [0 10]
      | dataSet.name = 'Group 1'
      | sbobj.Groups.Name = 'Group 1'
      | sbobj.Groups.Signals.Name = 'Signal 1'
      | sbobj.Groups.Signals.XData = [0 4 4 6 6 10]
      | sbobj.Groups.Signals.YData = [0 0 1 1 0 0]
  Signal 1 : Outport  Tag=STV Outport
  wires:
  Demux/1 -> Signal 1/1
  FromWs/1 -> Demux/1

== system sampleModel2438_pp/cfblk170 ==
  Demux : Demux  Tag=STV Demux  Outputs=1
  FromWs : FromWorkspace  Tag=STV FromWs  VariableName=tuvar  SampleTime=0
      SigBuilderData=|
      | common.afterFinalStr = 'Extrapolate'
      | common.sampleTime = 0
      | dataSet.timeRange = [0 10]
      | dataSet.name = 'Group 1'
      | sbobj.Groups.Name = 'Group 1'
      | sbobj.Groups.Signals.Name = 'Signal 1'
      | sbobj.Groups.Signals.XData = [0 4 4 6 6 10]
      | sbobj.Groups.Signals.YData = [0 0 1 1 0 0]
  Signal 1 : Outport  Tag=STV Outport
  wires:
  Demux/1 -> Signal 1/1
  FromWs/1 -> Demux/1

== system sampleModel2438_pp/cfblk179 ==
  Demux : Demux  Tag=STV Demux  Outputs=1
  FromWs : FromWorkspace  Tag=STV FromWs  VariableName=tuvar  SampleTime=0
      SigBuilderData=|
      | common.afterFinalStr = 'Extrapolate'
      | common.sampleTime = 0
      | dataSet.timeRange = [0 10]
      | dataSet.name = 'Group 1'
      | sbobj.Groups.Name = 'Group 1'
      | sbobj.Groups.Signals.Name = 'Signal 1'
      | sbobj.Groups.Signals.XData = [0 4 4 6 6 10]
      | sbobj.Groups.Signals.YData = [0 0 1 1 0 0]
  Signal 1 : Outport  Tag=STV Outport
  wires:
  Demux/1 -> Signal 1/1
  FromWs/1 -> Demux/1

== system sampleModel2438_pp/cfblk207 ==
  Demux : Demux  Tag=STV Demux  Outputs=1
  FromWs : FromWorkspace  Tag=STV FromWs  VariableName=tuvar  SampleTime=0
      SigBuilderData=|
      | common.afterFinalStr = 'Extrapolate'
      | common.sampleTime = 0
      | dataSet.timeRange = [0 10]
      | dataSet.name = 'Group 1'
      | sbobj.Groups.Name = 'Group 1'
      | sbobj.Groups.Signals.Name = 'Signal 1'
      | sbobj.Groups.Signals.XData = [0 4 4 6 6 10]
      | sbobj.Groups.Signals.YData = [0 0 1 1 0 0]
  Signal 1 : Outport  Tag=STV Outport
  wires:
  Demux/1 -> Signal 1/1
  FromWs/1 -> Demux/1

== system sampleModel2438_pp/cfblk230 ==
  cfblk1 : Inport
  cfblk13 : Inport  Port=2
  cfblk14 : Inport  Port=3
  Action Port : ActionPort  ActionType=then
  cfblk10 : UnitDelay  SampleTime=-1
  cfblk11 : DiscreteIntegrator  SampleTime=-1  ICPrevOutput=DiscIntNeverNeededParam  ICPrevScaledInput=DiscIntNeverNeededParam
  cfblk12 : simulink/Discrete/Transfer Fcn Lead or Lag  PoleZ=0.95  ZeroZ=0.75  ICPrevOutput=0.0  ICPrevInput=0.0  DoSatur=off
      settings: SourceProductName=Simulink  SourceProductBaseCode=SL
  cfblk15 : Delay
  cfblk3 : Delay  ShowEnablePort=on
      settings: InputPortMap=u0,e6
  cfblk4 : Delay
  cfblk5 : DiscreteFilter
  cfblk6 : Delay  DelayLengthSource=Input port
      settings: InputPortMap=u0,p1
  cfblk7 : DiscreteZeroPole  Poles=[0 0.5]  Gain=1  SampleTime=-1
  cfblk8 : DiscreteZeroPole  Poles=[0 0.5]  Gain=1  SampleTime=-1
  cfblk9 : UnitDelay  SampleTime=-1
  cyemi_{59..71} (13 alike) : DataTypeConversion  OutDataTypeStr=double
  cfblk2 : Outport
  wires:
  cfblk7/1 -> cfblk2/1
  cyemi_59/1 -> cfblk10/1
  cfblk8/1 -> cyemi_59/1
  cyemi_60/1 -> cfblk11/1
  cfblk10/1 -> cyemi_60/1
  cyemi_61/1 -> cfblk12/1
  cfblk4/1 -> cyemi_61/1
  cyemi_62/1 -> cfblk15/1
  cfblk9/1 -> cyemi_62/1
  cyemi_63/1 -> cfblk3/1
  cfblk6/1 -> cyemi_63/1
  cyemi_64/1 -> cfblk3/2
  cfblk15/1 -> cyemi_64/1
  cyemi_65/1 -> cfblk4/1
  cfblk1/1 -> cyemi_65/1
  cyemi_66/1 -> cfblk5/1
  cfblk12/1 -> cyemi_66/1
  cyemi_67/1 -> cfblk6/1
  cfblk5/1 -> cyemi_67/1
  cyemi_68/1 -> cfblk6/2
  cfblk13/1 -> cyemi_68/1
  cyemi_69/1 -> cfblk7/1
  cfblk11/1 -> cyemi_69/1
  cyemi_70/1 -> cfblk8/1
  cfblk14/1 -> cyemi_70/1
  cyemi_71/1 -> cfblk9/1
  cfblk3/1 -> cyemi_71/1

== system sampleModel2438_pp/cfblk231 ==
  cfblk1 : Inport
  Action Port : ActionPort  ActionType=else
  cfblk10 : Delay
  cfblk3 : simulink/Discrete/Difference  ICPrevInput=0.0  OutMin=[]  OutMax=[]  OutDataTypeStr=Inherit: Inherit via back propagation  OutDataType=fixdt(1, 16)  OutScaling=2^-10  DoSatur=off
  cfblk4 : DiscreteIntegrator  SampleTime=-1  ICPrevOutput=DiscIntNeverNeededParam  ICPrevScaledInput=DiscIntNeverNeededParam
  cfblk5 : Delay  ShowEnablePort=on
      settings: InputPortMap=u0,e6
  cfblk6 : Delay  ShowEnablePort=on
      settings: InputPortMap=u0,e6
  cfblk7 : DiscreteTransferFcn
  cfblk8 : Delay
  cfblk9 : DiscreteStateSpace  SampleTime=-1
  cyemi_{73..82} (10 alike) : DataTypeConversion  OutDataTypeStr=double
  cfblk2 : Outport
  wires:
  cfblk6/1 -> cfblk2/1
  cfblk1/1 -> cyemi_75/1, cyemi_78/1, cyemi_80/1
  cyemi_73/1 -> cfblk10/1
  cfblk8/1 -> cyemi_73/1
  cyemi_74/1 -> cfblk3/1
  cfblk4/1 -> cyemi_74/1
  cyemi_75/1 -> cfblk4/1
  cyemi_76/1 -> cfblk5/1
  cfblk10/1 -> cyemi_76/1
  cyemi_77/1 -> cfblk5/2
  cfblk9/1 -> cyemi_77/1
  cyemi_78/1 -> cfblk6/1
  cyemi_79/1 -> cfblk6/2
  cfblk3/1 -> cyemi_79/1
  cyemi_80/1 -> cfblk7/1
  cyemi_81/1 -> cfblk8/1
  cfblk5/1 -> cyemi_81/1
  cyemi_82/1 -> cfblk9/1
  cfblk7/1 -> cyemi_82/1

== system sampleModel2438_pp/cfblk232 ==
  cfblk1 : Inport
  cfblk8 : Inport  Port=2
  Action Port : ActionPort  ActionType=then
  cfblk10 : Subsystem  TreatAsAtomicUnit=on
  cfblk11 : Delay
  cfblk12 : Delay
  cfblk3 : Delay
  cfblk4 : simulink/Discrete/Transfer Fcn Lead or Lag  PoleZ=0.95  ZeroZ=0.75  ICPrevOutput=0.0  ICPrevInput=0.0  DoSatur=off
      settings: SourceProductName=Simulink  SourceProductBaseCode=SL
  cfblk5 : simulink/Discrete/Tapped Delay  vinit=0.0  samptime=-1  NumDelays=1  DelayOrder=Oldest  includeCurrent=off
  cfblk6 : simulink/Discrete/Tapped Delay  vinit=0.0  samptime=-1  NumDelays=1  DelayOrder=Oldest  includeCurrent=off
  cfblk7 : If  SampleTime=1
  cfblk9 : Subsystem  TreatAsAtomicUnit=on
  cyemi_{85..87,94..103} (13 alike) : DataTypeConversion  OutDataTypeStr=double
  cfblk2 : Outport
  wires:
  cfblk4/1 -> cfblk2/1
  cfblk7/1 -> cfblk9/Action
  cfblk7/2 -> cfblk10/Action
  cyemi_85/1 -> cfblk10/1(cfblk1)
  cfblk9/2(cfblk11) -> cyemi_85/1
  cyemi_86/1 -> cfblk10/2(cfblk8)
  cfblk9/3(cfblk12) -> cyemi_86/1, cyemi_87/1
  cyemi_87/1 -> cfblk10/3(cfblk9)
  cyemi_94/1 -> cfblk11/1
  cfblk10/1(cfblk2) -> cyemi_94/1
  cyemi_95/1 -> cfblk12/1
  cfblk5/1 -> cyemi_95/1
  cyemi_96/1 -> cfblk3/1
  cfblk9/1(cfblk2) -> cyemi_96/1
  cyemi_97/1 -> cfblk4/1
  cfblk3/1 -> cyemi_97/1
  cyemi_98/1 -> cfblk5/1
  cfblk6/1 -> cyemi_98/1
  cyemi_99/1 -> cfblk6/1
  cfblk10/2(cfblk10) -> cyemi_99/1
  cyemi_100/1 -> cfblk7/1
  cfblk8/1 -> cyemi_100/1
  cyemi_101/1 -> cfblk9/1(cfblk1)
  cfblk12/1 -> cyemi_101/1
  cyemi_102/1 -> cfblk9/2(cfblk9)
  cfblk1/1 -> cyemi_102/1
  cyemi_103/1 -> cfblk9/3(cfblk10)
  cfblk11/1 -> cyemi_103/1

== system sampleModel2438_pp/cfblk233 ==
  cfblk1 : Inport
  cfblk13 : Inport  Port=2
  cfblk14 : Inport  Port=3
  Action Port : ActionPort  ActionType=else
  cfblk10 : DiscreteStateSpace  SampleTime=-1
  cfblk11 : simulink/Discrete/Tapped Delay  vinit=0.0  samptime=-1  NumDelays=1  DelayOrder=Oldest  includeCurrent=off
  cfblk12 : simulink/Discrete/Transfer Fcn First Order  PoleZ=0.95  ICPrevOutput=0.0  DoSatur=off
      settings: SourceProductName=Simulink
  cfblk16 : Delay
  cfblk17 : Delay
  cfblk3 : DiscreteZeroPole  Poles=[0 0.5]  Gain=1  SampleTime=-1
  cfblk4 : Delay  DelayLengthSource=Input port
      settings: InputPortMap=u0,p1
  cfblk5 : Delay
  cfblk6 : Delay  ShowEnablePort=on
      settings: InputPortMap=u0,e6
  cfblk7 : DiscreteIntegrator  SampleTime=-1  ICPrevOutput=DiscIntNeverNeededParam  ICPrevScaledInput=DiscIntNeverNeededParam
  cfblk8 : simulink/Discrete/Transfer Fcn First Order  PoleZ=0.95  ICPrevOutput=0.0  DoSatur=off
      settings: SourceProductName=Simulink
  cfblk9 : DiscreteTransferFcn
  cyemi_{114..127} (14 alike) : DataTypeConversion  OutDataTypeStr=double
  cfblk2 : Outport
  cfblk15 : Outport  Port=2
  wires:
  cfblk11/1 -> cfblk15/1
  cfblk8/1 -> cyemi_117/1, cyemi_127/1
  cfblk1/1 -> cfblk2/1
  cyemi_114/1 -> cfblk10/1
  cfblk5/1 -> cyemi_114/1
  cyemi_115/1 -> cfblk11/1
  cfblk9/1 -> cyemi_115/1
  cyemi_116/1 -> cfblk12/1
  cfblk14/1 -> cyemi_116/1
  cyemi_117/1 -> cfblk16/1
  cyemi_118/1 -> cfblk17/1
  cfblk7/1 -> cyemi_118/1
  cyemi_119/1 -> cfblk3/1
  cfblk10/1 -> cyemi_119/1
  cyemi_120/1 -> cfblk4/1
  cfblk17/1 -> cyemi_120/1
  cyemi_121/1 -> cfblk4/2
  cfblk12/1 -> cyemi_121/1
  cyemi_122/1 -> cfblk5/1
  cfblk13/1 -> cyemi_122/1
  cyemi_123/1 -> cfblk6/1
  cfblk3/1 -> cyemi_123/1
  cyemi_124/1 -> cfblk6/2
  cfblk16/1 -> cyemi_124/1
  cyemi_125/1 -> cfblk7/1
  cfblk4/1 -> cyemi_125/1
  cyemi_126/1 -> cfblk8/1
  cfblk6/1 -> cyemi_126/1
  cyemi_127/1 -> cfblk9/1

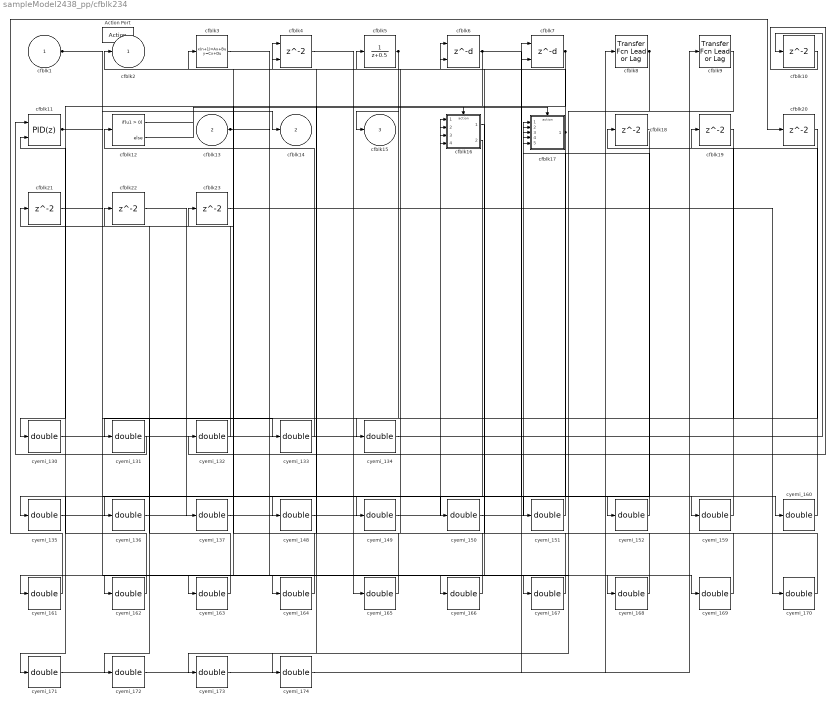
== system sampleModel2438_pp/cfblk234 ==
  cfblk1 : Inport
  cfblk13 : Inport  Port=2
  Action Port : ActionPort  ActionType=then
  cfblk{10,18..23} (7 alike) : Delay
  cfblk11 : simulink/Continuous/PID Controller (2DOF)  Controller=PID  TimeDomain=Discrete-time  SampleTime=-1  IntegratorMethod=Forward Euler  FilterMethod=Forward Euler  Form=Parallel  UseFilter=on  ControllerParametersSource=internal  P=1  I=1  D=0  N=100  b=1  c=1  InitialConditionSource=internal  InitialConditionForIntegrator=0  InitialConditionForFilter=0  ExternalReset=none  LimitOutput=off  UpperSaturationLimit=inf  LowerSaturationLimit=-inf  LinearizeAsGain=off  AntiWindupMode=none  Kb=1  TrackingMode=off  Kt=1  PParamMin=[]  PParamMax=[]  IParamMin=[]  IParamMax=[]  DParamMin=[]  DParamMax=[]  NParamMin=[]  NParamMax=[]  bParamMin=[]  bParamMax=[]  cParamMin=[]  cParamMax=[]  KbParamMin=[]  KbParamMax=[]  KtParamMin=[]  KtParamMax=[]  POutMin=[]  POutMax=[]  IOutMin=[]  IOutMax=[]  DOutMin=[]  DOutMax=[]  NOutMin=[]  NOutMax=[]  bOutMin=[]  bOutMax=[]  cOutMin=[]  cOutMax=[]  KbOutMin=[]  KbOutMax=[]  KtOutMin=[]  KtOutMax=[]  IntegratorOutMin=[]  IntegratorOutMax=[]  FilterOutMin=[]  FilterOutMax=[]  SumOutMin=[]  SumOutMax=[]  Sum1OutMin=[]  Sum1OutMax=[]  Sum2OutMin=[]  Sum2OutMax=[]  Sum3OutMin=[]  Sum3OutMax=[]  SumI1OutMin=[]  SumI1OutMax=[]  SumI2OutMin=[]  SumI2OutMax=[]  SumI3OutMin=[]  SumI3OutMax=[]  SumDOutMin=[]  SumDOutMax=[]  SaturationOutMin=[]  SaturationOutMax=[]  IntegratorContinuousStateAttributes=''  IntegratorStateMustResolveToSignalObject=off  IntegratorRTWStateStorageClass=Auto  FilterContinuousStateAttributes=''  FilterStateMustResolveToSignalObject=off  FilterRTWStateStorageClass=Auto  DifferentiatorICPrevScaledInput=0  DifferentiatorOutMin=[]  DifferentiatorOutMax=[]  FilterDiffOutCoefMin=[]  FilterDiffOutCoefMax=[]  SumDenOutMin=[]  SumDenOutMax=[]  SumNumOutMin=[]  SumNumOutMax=[]  ReciprocalOutMin=[]  ReciprocalOutMax=[]  DivideOutMin=[]  DivideOutMax=[]  TunerSelectOption=Transfer Function Based (PID Tuner App)
  cfblk12 : If  SampleTime=1
  cfblk16 : Subsystem  TreatAsAtomicUnit=on
  cfblk17 : Subsystem  TreatAsAtomicUnit=on
  cfblk3 : DiscreteStateSpace  SampleTime=-1
  cfblk4 : Delay  ShowEnablePort=on
      settings: InputPortMap=u0,e6
  cfblk5 : DiscreteTransferFcn
  cfblk6 : Delay  DelayLengthSource=Input port
      settings: InputPortMap=u0,p1
  cfblk7 : Delay  DelayLengthSource=Input port
      settings: InputPortMap=u0,p1
  cfblk8 : simulink/Discrete/Transfer Fcn Lead or Lag  PoleZ=0.95  ZeroZ=0.75  ICPrevOutput=0.0  ICPrevInput=0.0  DoSatur=off
      settings: SourceProductName=Simulink  SourceProductBaseCode=SL
  cfblk9 : simulink/Discrete/Transfer Fcn Lead or Lag  PoleZ=0.95  ZeroZ=0.75  ICPrevOutput=0.0  ICPrevInput=0.0  DoSatur=off
      settings: SourceProductName=Simulink  SourceProductBaseCode=SL
  cyemi_{130..137,148..152,159..174} (29 alike) : DataTypeConversion  OutDataTypeStr=double
  cfblk2 : Outport
  cfblk14 : Outport  Port=2
  cfblk15 : Outport  Port=3
  wires:
  cfblk6/1 -> cyemi_152/1, cyemi_174/1
  cfblk17/1(cfblk2) -> cfblk2/1, cyemi_171/1
  cfblk8/1 -> cyemi_135/1, cyemi_148/1, cyemi_151/1, cyemi_164/1, cyemi_167/1
  cfblk7/1 -> cyemi_130/1, cyemi_163/1
  cfblk13/1 -> cyemi_150/1, cyemi_166/1
  cfblk1/1 -> cfblk14/1, cyemi_169/1
  cfblk5/1 -> cfblk15/1, cyemi_136/1, cyemi_172/1
  cfblk11/1 -> cyemi_159/1, cyemi_160/1
  cfblk12/1 -> cfblk16/Action
  cfblk12/2 -> cfblk17/Action
  cyemi_130/1 -> cfblk10/1
  cyemi_131/1 -> cfblk11/1
  cfblk20/1 -> cyemi_131/1
  cyemi_132/1 -> cfblk11/2
  cfblk10/1 -> cyemi_132/1
  cyemi_133/1 -> cfblk12/1
  cfblk21/1 -> cyemi_133/1
  cyemi_134/1 -> cfblk16/1(cfblk1)
  cfblk19/1 -> cyemi_134/1
  cyemi_135/1 -> cfblk16/2(cfblk11)
  cyemi_136/1 -> cfblk16/3(cfblk12)
  cyemi_137/1 -> cfblk16/4(cfblk13)
  cfblk22/1 -> cyemi_137/1
  cyemi_148/1 -> cfblk17/1(cfblk1)
  cyemi_149/1 -> cfblk17/2(cfblk9)
  cfblk18/1 -> cyemi_149/1
  cyemi_150/1 -> cfblk17/3(cfblk10)
  cyemi_151/1 -> cfblk17/4(cfblk11)
  cyemi_152/1 -> cfblk17/5(cfblk12)
  cyemi_159/1 -> cfblk18/1
  cyemi_160/1 -> cfblk19/1
  cyemi_161/1 -> cfblk20/1
  cfblk16/1(cfblk2) -> cyemi_161/1
  cyemi_162/1 -> cfblk21/1
  cfblk16/2(cfblk14) -> cyemi_162/1
  cyemi_163/1 -> cfblk22/1
  cyemi_164/1 -> cfblk23/1
  cyemi_165/1 -> cfblk3/1
  cfblk4/1 -> cyemi_165/1
  cyemi_166/1 -> cfblk4/1
  cyemi_167/1 -> cfblk4/2
  cyemi_168/1 -> cfblk5/1
  cfblk3/1 -> cyemi_168/1
  cyemi_169/1 -> cfblk6/1
  cyemi_170/1 -> cfblk6/2
  cfblk23/1 -> cyemi_170/1
  cyemi_171/1 -> cfblk7/1
  cyemi_172/1 -> cfblk7/2
  cyemi_173/1 -> cfblk8/1
  cfblk9/1 -> cyemi_173/1
  cyemi_174/1 -> cfblk9/1
